simulink model "question_2"  (R2019a)
settings: Solver=ode4  StartTime=0.0  StopTime=50.0  FixedStep=0.001  RelTol=1e-3
libraries: dspsrcs4 x1
settings Model: Creator=guima  LastModifiedBy=guima

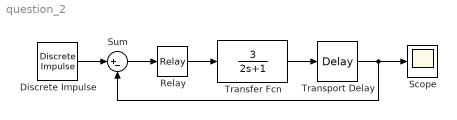
== system question_2 ==
  Discrete Impulse : dspsrcs4/Discrete  Impulse  Delay=0  SampleTime=0.001  FrameSample=1  OutputFrames=off  dataType=double  isSigned=on  wordLen=16  udDataType=sfix(16)  fracBitsMode=Best precision  numFracBits=15  OutDataTypeStr=double  LastOutDataTypeStr=double
  Relay : Relay  OnSwitchValue=0.1  OffSwitchValue=-0.1  OnOutputValue=5  OffOutputValue=-5
  Scope : Scope
  Sum : Sum  Inputs=|+-
  Transfer Fcn : TransferFcn  Numerator=[3]  Denominator=[2 1]
  Transport Delay : TransportDelay  DelayTime=0.1
  wires:
  Sum/1 -> Relay/1
  Relay/1 -> Transfer Fcn/1
  Discrete Impulse/1 -> Sum/1
  Transfer Fcn/1 -> Transport Delay/1
  Transport Delay/1 -> Scope/1, Sum/2
